simulink model "platooning_multiple_followers"  (R2018a)
settings: Solver=FixedStepAuto  StartTime=0.0  StopTime=70  FixedStep=timestep  RelTol=1e-3
model workspace (MAT data in the model file):
  t_0 = 0
undefined symbols (not defined in the file): a_max, a_min, canChannel, follower_1, follower_2, follower_3, leader, N
libraries: canlib x16, canmsglib x15, dspstat3 x3, dspindex x3, simulink x1
(part 1 of 2)
settings Model: Creator=s132652  LastModifiedBy=hugo
settings CodeAppCC: StateflowObjectComments=on
settings SimscapeCC: SimscapeNormalizeSystem=off

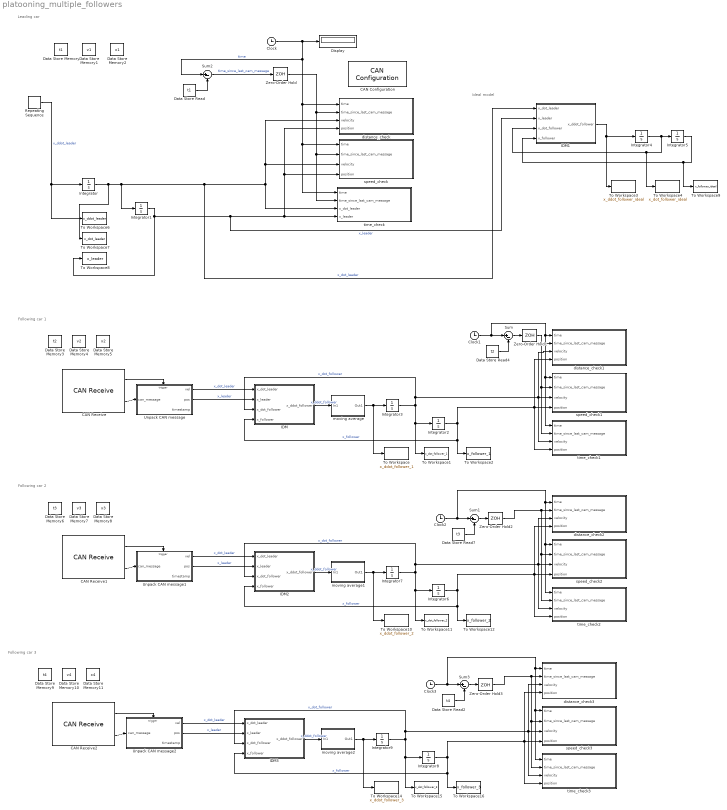
== system platooning_multiple_followers ==
  note: Ideal model
  note: Leading car
  note: Following car 1
  note: Following car 2
  note: Following car 3
  CAN Configuration : canlib/CAN Configuration  BlockHandle=4.0002  DeviceMenu=MathWorks Virtual 1 (Channel 1)  Device=MathWorks Virtual 1 (Channel 1)  ObjConstructor=canChannel('MathWorks','Virtual 1',1)  BusSpeed=500000  EnableBitParameters=off  SJW=0  TSEG1=0  TSEG2=0  NSamples=0  AckMode=Normal
      settings: SourceProductName=Vehicle Network Toolbox  SourceProductBaseCode=VN
  CAN Receive : canlib/CAN Receive  BlockHandle=5.0002  DeviceMenu=MathWorks Virtual 1 (Channel 1)  Device=MathWorks Virtual 1 (Channel 1)  ObjConstructor=canChannel('MathWorks','Virtual 1',1)  EnableStandardIDsFilter=off  StandardIDs=1  EnableExtendedIDsFilter=off  ExtendedIDs=0  SampleTime=0.001  MsgsPerTimestep=all  StdIDsCombo=Allow only  ExtIDsCombo=Allow all  InternalFilterUpdateStatus=on  BusOutput=off
      settings: SourceProductName=Vehicle Network Toolbox  SourceProductBaseCode=VN
  CAN Receive1 : canlib/CAN Receive  BlockHandle=6.0002  DeviceMenu=MathWorks Virtual 1 (Channel 1)  Device=MathWorks Virtual 1 (Channel 1)  ObjConstructor=canChannel('MathWorks','Virtual 1',1)  EnableStandardIDsFilter=off  StandardIDs=2  EnableExtendedIDsFilter=off  ExtendedIDs=0  SampleTime=0.001  MsgsPerTimestep=all  StdIDsCombo=Allow only  ExtIDsCombo=Allow all  InternalFilterUpdateStatus=on  BusOutput=off
      settings: SourceProductName=Vehicle Network Toolbox  SourceProductBaseCode=VN
  CAN Receive2 : canlib/CAN Receive  BlockHandle=7.0002  DeviceMenu=MathWorks Virtual 1 (Channel 1)  Device=MathWorks Virtual 1 (Channel 1)  ObjConstructor=canChannel('MathWorks','Virtual 1',1)  EnableStandardIDsFilter=off  StandardIDs=3  EnableExtendedIDsFilter=off  ExtendedIDs=0  SampleTime=0.001  MsgsPerTimestep=all  StdIDsCombo=Allow only  ExtIDsCombo=Allow all  InternalFilterUpdateStatus=on  BusOutput=off
      settings: SourceProductName=Vehicle Network Toolbox  SourceProductBaseCode=VN
  Clock{,1..3} (4 alike) : Clock
  Data Store Memory : DataStoreMemory  DataStoreName=t1  ReadBeforeWriteMsg=warning  WriteAfterWriteMsg=warning  WriteAfterReadMsg=warning  ShowAdditionalParam=off
  Data Store Memory1 : DataStoreMemory  DataStoreName=v1  ReadBeforeWriteMsg=warning  WriteAfterWriteMsg=warning  WriteAfterReadMsg=warning  InitialValue=leader.v0  ShowAdditionalParam=off
  Data Store Memory10 : DataStoreMemory  DataStoreName=v4  ReadBeforeWriteMsg=warning  WriteAfterWriteMsg=warning  WriteAfterReadMsg=warning  InitialValue=follower_3.v0  ShowAdditionalParam=off
  Data Store Memory11 : DataStoreMemory  DataStoreName=x4  ReadBeforeWriteMsg=warning  WriteAfterWriteMsg=warning  WriteAfterReadMsg=warning  InitialValue=follower_3.x0  ShowAdditionalParam=off
  Data Store Memory2 : DataStoreMemory  DataStoreName=x1  ReadBeforeWriteMsg=warning  WriteAfterWriteMsg=warning  WriteAfterReadMsg=warning  InitialValue=leader.x0  ShowAdditionalParam=off
  Data Store Memory3 : DataStoreMemory  DataStoreName=t2  ReadBeforeWriteMsg=warning  WriteAfterWriteMsg=warning  WriteAfterReadMsg=warning  ShowAdditionalParam=off
  Data Store Memory4 : DataStoreMemory  DataStoreName=v2  ReadBeforeWriteMsg=warning  WriteAfterWriteMsg=warning  WriteAfterReadMsg=warning  InitialValue=follower_1.v0  ShowAdditionalParam=off
  Data Store Memory5 : DataStoreMemory  DataStoreName=x2  ReadBeforeWriteMsg=warning  WriteAfterWriteMsg=warning  WriteAfterReadMsg=warning  InitialValue=follower_1.x0  ShowAdditionalParam=off
  Data Store Memory6 : DataStoreMemory  DataStoreName=t3  ReadBeforeWriteMsg=warning  WriteAfterWriteMsg=warning  WriteAfterReadMsg=warning  ShowAdditionalParam=off
  Data Store Memory7 : DataStoreMemory  DataStoreName=v3  ReadBeforeWriteMsg=warning  WriteAfterWriteMsg=warning  WriteAfterReadMsg=warning  InitialValue=follower_2.v0  ShowAdditionalParam=off
  Data Store Memory8 : DataStoreMemory  DataStoreName=x3  ReadBeforeWriteMsg=warning  WriteAfterWriteMsg=warning  WriteAfterReadMsg=warning  InitialValue=follower_2.x0  ShowAdditionalParam=off
  Data Store Memory9 : DataStoreMemory  DataStoreName=t4  ReadBeforeWriteMsg=warning  WriteAfterWriteMsg=warning  WriteAfterReadMsg=warning  ShowAdditionalParam=off
  Data Store Read : DataStoreRead  DataStoreName=t1
  Data Store Read2 : DataStoreRead  DataStoreName=t4
  Data Store Read4 : DataStoreRead  DataStoreName=t2
  Data Store Read7 : DataStoreRead  DataStoreName=t3
  Display : Display
  IDM : Subsystem
  IDM1 : Subsystem
  IDM2 : Subsystem
  IDM3 : Subsystem
  Integrator : Integrator  InitialCondition=leader.v0
  Integrator1 : Integrator  InitialCondition=leader.x0
  Integrator2 : Integrator  InitialCondition=follower_1.x0
  Integrator3 : Integrator  InitialCondition=follower_1.v0
  Integrator4 : Integrator  InitialCondition=follower_1.v0
  Integrator5 : Integrator  InitialCondition=follower_1.x0
  Integrator6 : Integrator  InitialCondition=follower_2.x0
  Integrator7 : Integrator  InitialCondition=follower_2.v0
  Integrator8 : Integrator  InitialCondition=follower_3.x0
  Integrator9 : Integrator  InitialCondition=follower_3.v0
  Repeating Sequence : simulink/Sources/Repeating Sequence  rep_seq_t=[0 5 10 15 20 25 30 35 40 45 50 55 60 65 70]  rep_seq_y=[0 0 0 0 0 a_max a_max 0 0 0 a_min a_min 0 0 0]
  Sum{,1..3} (4 alike) : Sum  Inputs=|+-
  To Workspace : ToWorkspace  VariableName=x_ddot_follower_1  SaveFormat=Timeseries  SampleTime=-1
  To Workspace1 : ToWorkspace  VariableName=x_dot_follower_1  SaveFormat=Timeseries  SampleTime=-1
  To Workspace10 : ToWorkspace  VariableName=x_ddot_follower_2  SaveFormat=Timeseries  SampleTime=-1
  To Workspace11 : ToWorkspace  VariableName=x_dot_follower_2  SaveFormat=Timeseries  SampleTime=-1
  To Workspace12 : ToWorkspace  VariableName=x_follower_2  SaveFormat=Timeseries  SampleTime=-1
  To Workspace14 : ToWorkspace  VariableName=x_ddot_follower_3  SaveFormat=Timeseries  SampleTime=-1
  To Workspace15 : ToWorkspace  VariableName=x_dot_follower_3  SaveFormat=Timeseries  SampleTime=-1
  To Workspace16 : ToWorkspace  VariableName=x_follower_3  SaveFormat=Timeseries  SampleTime=-1
  To Workspace2 : ToWorkspace  VariableName=x_follower_1  SaveFormat=Timeseries  SampleTime=-1
  To Workspace3 : ToWorkspace  VariableName=x_ddot_follower_ideal  SaveFormat=Timeseries  SampleTime=-1
  To Workspace4 : ToWorkspace  VariableName=x_dot_follower_ideal  SaveFormat=Timeseries  SampleTime=-1
  To Workspace6 : ToWorkspace  VariableName=x_ddot_leader  SaveFormat=Timeseries  SampleTime=-1
  To Workspace7 : ToWorkspace  VariableName=x_dot_leader  SaveFormat=Timeseries  SampleTime=-1
  To Workspace8 : ToWorkspace  VariableName=x_leader  SaveFormat=Timeseries  SampleTime=-1
  To Workspace9 : ToWorkspace  VariableName=x_follower_ideal  SaveFormat=Timeseries  SampleTime=-1
  Unpack CAN message : Subsystem  TreatAsAtomicUnit=on
  Unpack CAN message1 : Subsystem  TreatAsAtomicUnit=on
  Unpack CAN message2 : Subsystem  TreatAsAtomicUnit=on
  Zero-Order Hold{,1..3} (4 alike) : ZeroOrderHold  SampleTime=.001
  distance_check : Subsystem
  distance_check1 : Subsystem
  distance_check2 : Subsystem
  distance_check3 : Subsystem
  moving average : Subsystem
  moving average1 : Subsystem
  moving average2 : Subsystem
  speed_check : Subsystem
  speed_check1 : Subsystem
  speed_check2 : Subsystem
  speed_check3 : Subsystem
  time_check : Subsystem
  time_check1 : Subsystem
  time_check2 : Subsystem
  time_check3 : Subsystem
  wires:
  Repeating Sequence/1 -> To Workspace6/1, Integrator/1  "x_ddot_leader"
  Integrator/1 -> To Workspace7/1, Integrator1/1, IDM1/1(x_dot_leader), distance_check/3(velocity), speed_check/3(velocity), time_check/3(x_dot_leader)  "x_dot_leader"
  Integrator1/1 -> To Workspace8/1, IDM1/2(x_leader), distance_check/4(position), speed_check/4(position), time_check/4(x_leader)  "x_leader"
  Clock/1 -> time_check/1(time), speed_check/1(time), distance_check/1(time), Sum2/1, Display/1  "time"
  Data Store Read/1 -> Sum2/2
  Sum2/1 -> Zero-Order Hold/1  "time_since_last_cam_message"
  Zero-Order Hold/1 -> time_check/2(time_since_last_cam_message), speed_check/2(time_since_last_cam_message), distance_check/2(time_since_last_cam_message)
  CAN Receive/2 -> Unpack CAN message/1(can_message)
  CAN Receive/1 -> Unpack CAN message/Trigger
  Unpack CAN message/1(vel) -> IDM/1(x_dot_leader)  "x_dot_leader"
  Unpack CAN message/2(pos) -> IDM/2(x_leader)  "x_leader"
  IDM/1(x_ddot_follower) -> moving average/1(In1)  "x_ddot_follower"
  moving average/1(Out1) -> To Workspace/1, Integrator3/1
  Integrator3/1 -> speed_check1/3(velocity), distance_check1/3(velocity), time_check1/3(velocity), IDM/3(x_dot_follower), Integrator2/1, To Workspace1/1  "x_dot_follower"
  Integrator2/1 -> To Workspace2/1, IDM/4(x_follower), distance_check1/4(position), time_check1/4(position), speed_check1/4(position)  "x_follower"
  Integrator4/1 -> IDM1/3(x_dot_follower), To Workspace4/1, Integrator5/1
  Integrator5/1 -> IDM1/4(x_follower), To Workspace9/1
  IDM1/1(x_ddot_follower) -> Integrator4/1, To Workspace3/1
  Clock1/1 -> Sum/1, time_check1/1(time), speed_check1/1(time), distance_check1/1(time)
  Data Store Read4/1 -> Sum/2
  Sum/1 -> Zero-Order Hold1/1
  Zero-Order Hold1/1 -> time_check1/2(time_since_last_cam_message), speed_check1/2(time_since_last_cam_message), distance_check1/2(time_since_last_cam_message)
  Data Store Read7/1 -> Sum1/2
  Zero-Order Hold2/1 -> time_check2/2(time_since_last_cam_message), speed_check2/2(time_since_last_cam_message), distance_check2/2(time_since_last_cam_message)
  IDM2/1(x_ddot_follower) -> moving average1/1(In1)  "x_ddot_follower"
  Clock2/1 -> Sum1/1, time_check2/1(time), speed_check2/1(time), distance_check2/1(time)
  Integrator6/1 -> distance_check2/4(position), time_check2/4(position), speed_check2/4(position), To Workspace12/1, IDM2/4(x_follower)  "x_follower"
  Unpack CAN message1/2(pos) -> IDM2/2(x_leader)  "x_leader"
  Integrator7/1 -> speed_check2/3(velocity), distance_check2/3(velocity), time_check2/3(velocity), IDM2/3(x_dot_follower), Integrator6/1, To Workspace11/1  "x_dot_follower"
  moving average1/1(Out1) -> To Workspace10/1, Integrator7/1
  CAN Receive1/1 -> Unpack CAN message1/Trigger
  Unpack CAN message1/1(vel) -> IDM2/1(x_dot_leader)  "x_dot_leader"
  Sum1/1 -> Zero-Order Hold2/1
  CAN Receive1/2 -> Unpack CAN message1/1(can_message)
  Data Store Read2/1 -> Sum3/2
  CAN Receive2/1 -> Unpack CAN message2/Trigger
  IDM3/1(x_ddot_follower) -> moving average2/1(In1)  "x_ddot_follower"
  Sum3/1 -> Zero-Order Hold3/1
  CAN Receive2/2 -> Unpack CAN message2/1(can_message)
  Unpack CAN message2/1(vel) -> IDM3/1(x_dot_leader)  "x_dot_leader"
  Unpack CAN message2/2(pos) -> IDM3/2(x_leader)  "x_leader"
  Clock3/1 -> Sum3/1, time_check3/1(time), speed_check3/1(time), distance_check3/1(time)
  moving average2/1(Out1) -> To Workspace14/1, Integrator9/1
  Zero-Order Hold3/1 -> time_check3/2(time_since_last_cam_message), speed_check3/2(time_since_last_cam_message), distance_check3/2(time_since_last_cam_message)
  Integrator9/1 -> speed_check3/3(velocity), distance_check3/3(velocity), time_check3/3(velocity), IDM3/3(x_dot_follower), Integrator8/1, To Workspace15/1  "x_dot_follower"
  Integrator8/1 -> distance_check3/4(position), time_check3/4(position), speed_check3/4(position), To Workspace16/1, IDM3/4(x_follower)  "x_follower"

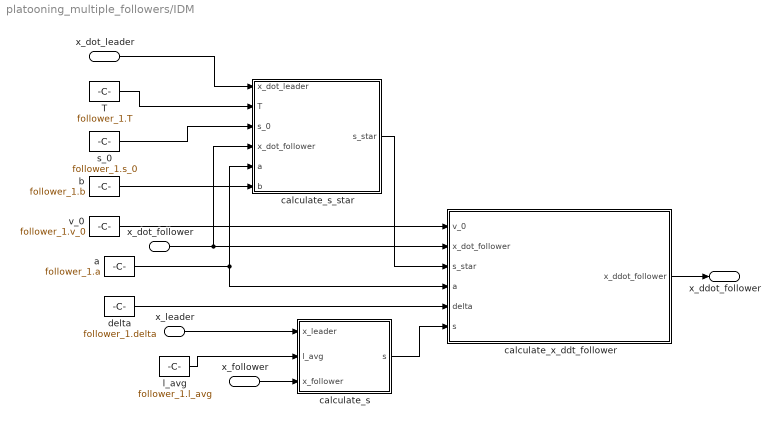
== system platooning_multiple_followers/IDM ==
  x_dot_leader : Inport
  x_leader : Inport  Port=2
  x_dot_follower : Inport  Port=3
  x_follower : Inport  Port=4
  T : Constant  Value=follower_1.T
  a : Constant  Value=follower_1.a
  b : Constant  Value=follower_1.b
  calculate_s : Subsystem
  calculate_s_star : Subsystem
  calculate_x_ddt_follower : Subsystem
  delta : Constant  Value=follower_1.delta
  l_avg : Constant  Value=follower_1.l_avg
  s_0 : Constant  Value=follower_1.s_0
  v_0 : Constant  Value=follower_1.v_0
  x_ddot_follower : Outport
  wires:
  v_0/1 -> calculate_x_ddt_follower/1(v_0)
  T/1 -> calculate_s_star/2(T)
  s_0/1 -> calculate_s_star/3(s_0)
  calculate_x_ddt_follower/1(x_ddot_follower) -> x_ddot_follower/1
  b/1 -> calculate_s_star/6(b)
  l_avg/1 -> calculate_s/2(l_avg)
  calculate_s/1(s) -> calculate_x_ddt_follower/6(s)
  delta/1 -> calculate_x_ddt_follower/5(delta)
  calculate_s_star/1(s_star) -> calculate_x_ddt_follower/3(s_star)
  x_follower/1 -> calculate_s/3(x_follower)
  x_dot_leader/1 -> calculate_s_star/1(x_dot_leader)
  x_leader/1 -> calculate_s/1(x_leader)
  x_dot_follower/1 -> calculate_s_star/4(x_dot_follower), calculate_x_ddt_follower/2(x_dot_follower)
  a/1 -> calculate_x_ddt_follower/4(a), calculate_s_star/5(a)

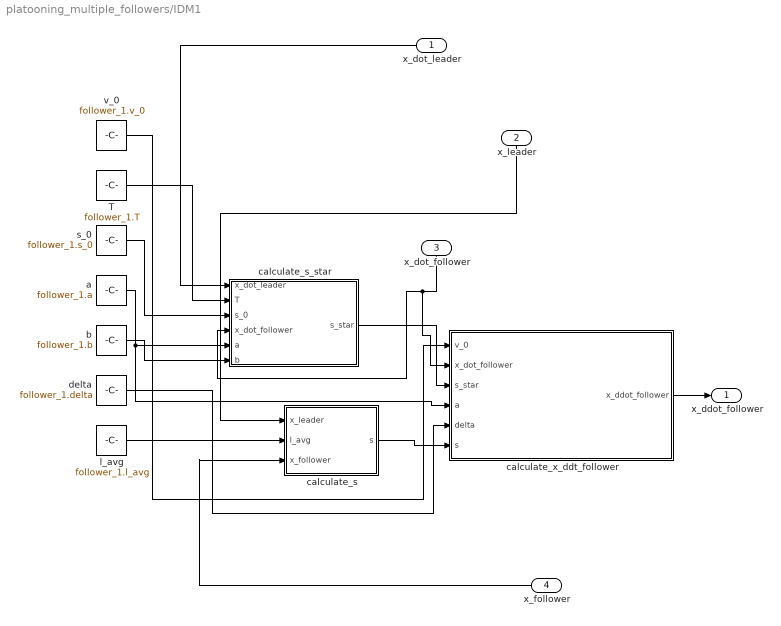
== system platooning_multiple_followers/IDM1 ==
  x_dot_leader : Inport
  x_leader : Inport  Port=2
  x_dot_follower : Inport  Port=3
  x_follower : Inport  Port=4
  T : Constant  Value=follower_1.T
  a : Constant  Value=follower_1.a
  b : Constant  Value=follower_1.b
  calculate_s : Subsystem
  calculate_s_star : Subsystem
  calculate_x_ddt_follower : Subsystem
  delta : Constant  Value=follower_1.delta
  l_avg : Constant  Value=follower_1.l_avg
  "s_0 " : Constant  Value=follower_1.s_0
  v_0 : Constant  Value=follower_1.v_0
  x_ddot_follower : Outport
  wires:
  a/1 -> calculate_x_ddt_follower/4(a), calculate_s_star/5(a)
  v_0/1 -> calculate_x_ddt_follower/1(v_0)
  T/1 -> calculate_s_star/2(T)
  "s_0 "/1 -> calculate_s_star/3(s_0)
  calculate_x_ddt_follower/1(x_ddot_follower) -> x_ddot_follower/1
  b/1 -> calculate_s_star/6(b)
  l_avg/1 -> calculate_s/2(l_avg)
  calculate_s/1(s) -> calculate_x_ddt_follower/6(s)
  delta/1 -> calculate_x_ddt_follower/5(delta)
  calculate_s_star/1(s_star) -> calculate_x_ddt_follower/3(s_star)
  x_follower/1 -> calculate_s/3(x_follower)
  x_dot_follower/1 -> calculate_x_ddt_follower/2(x_dot_follower), calculate_s_star/4(x_dot_follower)
  x_dot_leader/1 -> calculate_s_star/1(x_dot_leader)
  x_leader/1 -> calculate_s/1(x_leader)

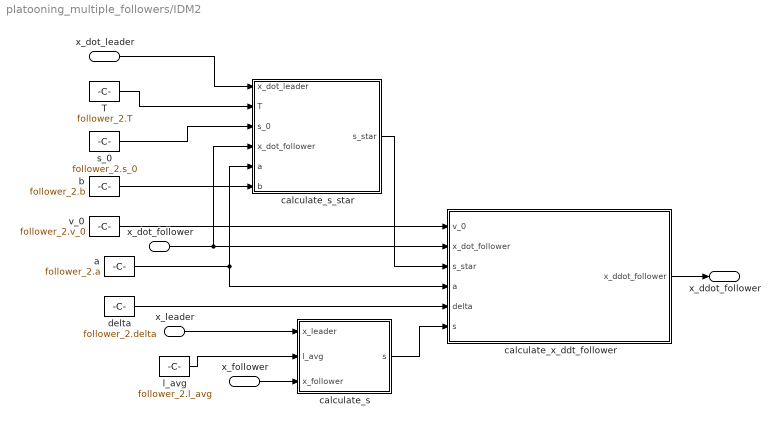
== system platooning_multiple_followers/IDM2 ==
  x_dot_leader : Inport
  x_leader : Inport  Port=2
  x_dot_follower : Inport  Port=3
  x_follower : Inport  Port=4
  T : Constant  Value=follower_2.T
  a : Constant  Value=follower_2.a
  b : Constant  Value=follower_2.b
  calculate_s : Subsystem
  calculate_s_star : Subsystem
  calculate_x_ddt_follower : Subsystem
  delta : Constant  Value=follower_2.delta
  l_avg : Constant  Value=follower_2.l_avg
  s_0 : Constant  Value=follower_2.s_0
  v_0 : Constant  Value=follower_2.v_0
  x_ddot_follower : Outport
  wires:
  v_0/1 -> calculate_x_ddt_follower/1(v_0)
  T/1 -> calculate_s_star/2(T)
  s_0/1 -> calculate_s_star/3(s_0)
  calculate_x_ddt_follower/1(x_ddot_follower) -> x_ddot_follower/1
  b/1 -> calculate_s_star/6(b)
  l_avg/1 -> calculate_s/2(l_avg)
  calculate_s/1(s) -> calculate_x_ddt_follower/6(s)
  delta/1 -> calculate_x_ddt_follower/5(delta)
  calculate_s_star/1(s_star) -> calculate_x_ddt_follower/3(s_star)
  x_follower/1 -> calculate_s/3(x_follower)
  x_dot_leader/1 -> calculate_s_star/1(x_dot_leader)
  x_leader/1 -> calculate_s/1(x_leader)
  x_dot_follower/1 -> calculate_s_star/4(x_dot_follower), calculate_x_ddt_follower/2(x_dot_follower)
  a/1 -> calculate_x_ddt_follower/4(a), calculate_s_star/5(a)

== system platooning_multiple_followers/IDM3 ==
  x_dot_leader : Inport
  x_leader : Inport  Port=2
  x_dot_follower : Inport  Port=3
  x_follower : Inport  Port=4
  T : Constant  Value=follower_3.T
  a : Constant  Value=follower_3.a
  b : Constant  Value=follower_3.b
  calculate_s : Subsystem
  calculate_s_star : Subsystem
  calculate_x_ddt_follower : Subsystem
  delta : Constant  Value=follower_3.delta
  l_avg : Constant  Value=follower_3.l_avg
  s_0 : Constant  Value=follower_3.s_0
  v_0 : Constant  Value=follower_3.v_0
  x_ddot_follower : Outport
  wires:
  v_0/1 -> calculate_x_ddt_follower/1(v_0)
  T/1 -> calculate_s_star/2(T)
  s_0/1 -> calculate_s_star/3(s_0)
  calculate_x_ddt_follower/1(x_ddot_follower) -> x_ddot_follower/1
  b/1 -> calculate_s_star/6(b)
  l_avg/1 -> calculate_s/2(l_avg)
  calculate_s/1(s) -> calculate_x_ddt_follower/6(s)
  delta/1 -> calculate_x_ddt_follower/5(delta)
  calculate_s_star/1(s_star) -> calculate_x_ddt_follower/3(s_star)
  x_follower/1 -> calculate_s/3(x_follower)
  x_dot_leader/1 -> calculate_s_star/1(x_dot_leader)
  x_leader/1 -> calculate_s/1(x_leader)
  x_dot_follower/1 -> calculate_s_star/4(x_dot_follower), calculate_x_ddt_follower/2(x_dot_follower)
  a/1 -> calculate_x_ddt_follower/4(a), calculate_s_star/5(a)

== system platooning_multiple_followers/Unpack CAN message ==
  can_message : Inport
  function : TriggerPort  TriggerType=function-call  VariantControl=Variant
  CAN Unpack : canmsglib/CAN Unpack  MsgList=(none)  MsgName=CAN Msg  MsgIDType=Standard (11-bit identifier)  MsgIdentifier=1  MsgLength=8  SignalInfo=position$0$16$1$1$1$0$0.1$0$-Inf$Inf$#velocity$16$16$1$1$1$0$0.0025$0$-Inf$Inf$#timestamp$32$16$1$1$1$0$0.01$0$-Inf$Inf$#  NSignals=3  IDPort=off  TimestampPort=off  ErrorPort=off  RemotePort=off  LengthPort=off  StatusPort=off  StartBits=str2num('[int32(0);int32(16);int32(32)]')  SignalSizes=str2num('[int32(16);int32(16);int32(16)]')  ByteOrders=str2num('[int32(1);int32(1);int32(1)]')  DataTypes=str2num('[int32(1);int32(1);int32(1)]')  MultiplexTypes=str2num('[int32(1);int32(1);int32(1)]')  MultiplexValues=str2num('[double(0);double(0);double(0)]')  Factors=str2num('[double(0.1);double(0.0025);double(0.01)]')  Offsets=str2num('[double(0);double(0);double(0)]')  Minimums=str2num('[double(-Inf);double(-Inf);double(-Inf)]')  Maximums=str2num('[double(Inf);double(Inf);double(Inf)]')  ApplyMinMax=off
      settings: SourceProductName=Simulink Real-Time
  vel : Outport
  pos : Outport  Port=2
  timestamp : Outport  Port=3
  wires:
  can_message/1 -> CAN Unpack/1
  CAN Unpack/2 -> vel/1
  CAN Unpack/1 -> pos/1
  CAN Unpack/3 -> timestamp/1

== system platooning_multiple_followers/Unpack CAN message1 ==
  can_message : Inport
  function : TriggerPort  TriggerType=function-call  VariantControl=Variant
  CAN Unpack : canmsglib/CAN Unpack  MsgList=(none)  MsgName=CAN Msg  MsgIDType=Standard (11-bit identifier)  MsgIdentifier=2  MsgLength=8  SignalInfo=position$0$16$1$1$1$0$0.1$0$-Inf$Inf$#velocity$16$16$1$1$1$0$0.0025$0$-Inf$Inf$#timestamp$32$16$1$1$1$0$0.01$0$-Inf$Inf$#  NSignals=3  IDPort=off  TimestampPort=off  ErrorPort=off  RemotePort=off  LengthPort=off  StatusPort=off  StartBits=str2num('[int32(0);int32(16);int32(32)]')  SignalSizes=str2num('[int32(16);int32(16);int32(16)]')  ByteOrders=str2num('[int32(1);int32(1);int32(1)]')  DataTypes=str2num('[int32(1);int32(1);int32(1)]')  MultiplexTypes=str2num('[int32(1);int32(1);int32(1)]')  MultiplexValues=str2num('[double(0);double(0);double(0)]')  Factors=str2num('[double(0.1);double(0.0025);double(0.01)]')  Offsets=str2num('[double(0);double(0);double(0)]')  Minimums=str2num('[double(-Inf);double(-Inf);double(-Inf)]')  Maximums=str2num('[double(Inf);double(Inf);double(Inf)]')  ApplyMinMax=off
      settings: SourceProductName=Simulink Real-Time
  vel : Outport
  pos : Outport  Port=2
  timestamp : Outport  Port=3
  wires:
  can_message/1 -> CAN Unpack/1
  CAN Unpack/2 -> vel/1
  CAN Unpack/1 -> pos/1
  CAN Unpack/3 -> timestamp/1

== system platooning_multiple_followers/Unpack CAN message2 ==
  can_message : Inport
  function : TriggerPort  TriggerType=function-call  VariantControl=Variant
  CAN Unpack : canmsglib/CAN Unpack  MsgList=(none)  MsgName=CAN Msg  MsgIDType=Standard (11-bit identifier)  MsgIdentifier=3  MsgLength=8  SignalInfo=position$0$16$1$1$1$0$0.1$0$-Inf$Inf$#velocity$16$16$1$1$1$0$0.0025$0$-Inf$Inf$#timestamp$32$16$1$1$1$0$0.01$0$-Inf$Inf$#  NSignals=3  IDPort=off  TimestampPort=off  ErrorPort=off  RemotePort=off  LengthPort=off  StatusPort=off  StartBits=str2num('[int32(0);int32(16);int32(32)]')  SignalSizes=str2num('[int32(16);int32(16);int32(16)]')  ByteOrders=str2num('[int32(1);int32(1);int32(1)]')  DataTypes=str2num('[int32(1);int32(1);int32(1)]')  MultiplexTypes=str2num('[int32(1);int32(1);int32(1)]')  MultiplexValues=str2num('[double(0);double(0);double(0)]')  Factors=str2num('[double(0.1);double(0.0025);double(0.01)]')  Offsets=str2num('[double(0);double(0);double(0)]')  Minimums=str2num('[double(-Inf);double(-Inf);double(-Inf)]')  Maximums=str2num('[double(Inf);double(Inf);double(Inf)]')  ApplyMinMax=off
      settings: SourceProductName=Simulink Real-Time
  vel : Outport
  pos : Outport  Port=2
  timestamp : Outport  Port=3
  wires:
  can_message/1 -> CAN Unpack/1
  CAN Unpack/2 -> vel/1
  CAN Unpack/1 -> pos/1
  CAN Unpack/3 -> timestamp/1

== system platooning_multiple_followers/distance_check ==
  time : Inport
  time_since_last_cam_message : Inport  Port=2
  velocity : Inport  Port=3
  position : Inport  Port=4
  Abs1 : Abs
  Data Store Read3 : DataStoreRead  DataStoreName=x1
  If Action Subsystem2 : Subsystem  TreatAsAtomicUnit=on
  If2 : If  NumInputs=2  IfExpression=u1 >= D_THRESHOLD & u2 >= 0.1
  Sum1 : Sum  Inputs=|+-
  Zero-Order Hold2 : ZeroOrderHold  SampleTime=.001
  wires:
  Data Store Read3/1 -> Sum1/2
  Sum1/1 -> Abs1/1
  Abs1/1 -> Zero-Order Hold2/1
  Zero-Order Hold2/1 -> If2/1
  If2/1 -> If Action Subsystem2/Action
  time_since_last_cam_message/1 -> If2/2
  time/1 -> If Action Subsystem2/1(time)
  position/1 -> If Action Subsystem2/3(position), Sum1/1
  velocity/1 -> If Action Subsystem2/2(velocity)

== system platooning_multiple_followers/distance_check1 ==
  time : Inport
  time_since_last_cam_message : Inport  Port=2
  velocity : Inport  Port=3
  position : Inport  Port=4
  Abs1 : Abs
  Data Store Read3 : DataStoreRead  DataStoreName=x2
  If Action Subsystem2 : Subsystem  TreatAsAtomicUnit=on
  If2 : If  NumInputs=2  IfExpression=u1 >= D_THRESHOLD & u2 >= 0.1
  Sum1 : Sum  Inputs=|+-
  Zero-Order Hold2 : ZeroOrderHold  SampleTime=.001
  wires:
  Data Store Read3/1 -> Sum1/2
  Sum1/1 -> Abs1/1
  Abs1/1 -> Zero-Order Hold2/1
  Zero-Order Hold2/1 -> If2/1
  If2/1 -> If Action Subsystem2/Action
  time_since_last_cam_message/1 -> If2/2
  time/1 -> If Action Subsystem2/1(time)
  position/1 -> If Action Subsystem2/3(position), Sum1/1
  velocity/1 -> If Action Subsystem2/2(velocity)

== system platooning_multiple_followers/distance_check2 ==
  time : Inport
  time_since_last_cam_message : Inport  Port=2
  velocity : Inport  Port=3
  position : Inport  Port=4
  Abs1 : Abs
  Data Store Read3 : DataStoreRead  DataStoreName=x3
  If Action Subsystem2 : Subsystem  TreatAsAtomicUnit=on
  If2 : If  NumInputs=2  IfExpression=u1 >= D_THRESHOLD & u2 >= 0.1
  Sum1 : Sum  Inputs=|+-
  Zero-Order Hold2 : ZeroOrderHold  SampleTime=.001
  wires:
  Data Store Read3/1 -> Sum1/2
  Sum1/1 -> Abs1/1
  Abs1/1 -> Zero-Order Hold2/1
  Zero-Order Hold2/1 -> If2/1
  If2/1 -> If Action Subsystem2/Action
  time_since_last_cam_message/1 -> If2/2
  time/1 -> If Action Subsystem2/1(time)
  position/1 -> If Action Subsystem2/3(position), Sum1/1
  velocity/1 -> If Action Subsystem2/2(velocity)

== system platooning_multiple_followers/distance_check3 ==
  time : Inport
  time_since_last_cam_message : Inport  Port=2
  velocity : Inport  Port=3
  position : Inport  Port=4
  Abs1 : Abs
  Data Store Read3 : DataStoreRead  DataStoreName=x4
  If Action Subsystem2 : Subsystem  TreatAsAtomicUnit=on
  If2 : If  NumInputs=2  IfExpression=u1 >= D_THRESHOLD & u2 >= 0.1
  Sum1 : Sum  Inputs=|+-
  Zero-Order Hold2 : ZeroOrderHold  SampleTime=.001
  wires:
  Data Store Read3/1 -> Sum1/2
  Sum1/1 -> Abs1/1
  Abs1/1 -> Zero-Order Hold2/1
  Zero-Order Hold2/1 -> If2/1
  If2/1 -> If Action Subsystem2/Action
  time_since_last_cam_message/1 -> If2/2
  time/1 -> If Action Subsystem2/1(time)
  position/1 -> If Action Subsystem2/3(position), Sum1/1
  velocity/1 -> If Action Subsystem2/2(velocity)

== system platooning_multiple_followers/moving average ==
  note: moving average
  In1 : Inport
  IC : InitialCondition  Value=zeros(N,1)
  Mean : dspstat3/Mean  run=off  InputProcessing=Columns as channels (frame based)  reset_popup=None  directionMode=Each column  dimension=1  roiEnable=off  roiType=Rectangles  roiPortion=Entire ROI  roiOutput=Individual statistics for each ROI  roiFlag=off  roundingMode=Floor  overflowMode=off  outputDataTypeStr=Inherit: Same as accumulator  outputMin=[]  outputMax=[]  outputLastDataTypeStr=Inherit: Same as accumulator
  Memory : Memory
  Mux : Mux  Inputs=2
  Variable Selector : dspindex/Variable Selector  NumInputs=1  rowsOrCols=Rows  IdxMode=Fixed  Elements=1:N-1  ZerOneIdxMode=One-based  errmode=Clip Index  FillMode=on  FillValues=0
  Out1 : Outport
  wires:
  In1/1 -> Mux/1
  Mux/1 -> Mean/1, Memory/1
  Memory/1 -> IC/1
  IC/1 -> Variable Selector/1
  Mean/1 -> Out1/1
  Variable Selector/1 -> Mux/2

== system platooning_multiple_followers/moving average1 ==
  note: moving average
  In1 : Inport
  IC : InitialCondition  Value=zeros(N,1)
  Mean : dspstat3/Mean  run=off  InputProcessing=Columns as channels (frame based)  reset_popup=None  directionMode=Each column  dimension=1  roiEnable=off  roiType=Rectangles  roiPortion=Entire ROI  roiOutput=Individual statistics for each ROI  roiFlag=off  roundingMode=Floor  overflowMode=off  outputDataTypeStr=Inherit: Same as accumulator  outputMin=[]  outputMax=[]  outputLastDataTypeStr=Inherit: Same as accumulator
  Memory : Memory
  Mux : Mux  Inputs=2
  Variable Selector : dspindex/Variable Selector  NumInputs=1  rowsOrCols=Rows  IdxMode=Fixed  Elements=1:N-1  ZerOneIdxMode=One-based  errmode=Clip Index  FillMode=on  FillValues=0
  Out1 : Outport
  wires:
  In1/1 -> Mux/1
  Mux/1 -> Mean/1, Memory/1
  Memory/1 -> IC/1
  IC/1 -> Variable Selector/1
  Mean/1 -> Out1/1
  Variable Selector/1 -> Mux/2

== system platooning_multiple_followers/moving average2 ==
  note: moving average
  In1 : Inport
  IC : InitialCondition  Value=zeros(N,1)
  Mean : dspstat3/Mean  run=off  InputProcessing=Columns as channels (frame based)  reset_popup=None  directionMode=Each column  dimension=1  roiEnable=off  roiType=Rectangles  roiPortion=Entire ROI  roiOutput=Individual statistics for each ROI  roiFlag=off  roundingMode=Floor  overflowMode=off  outputDataTypeStr=Inherit: Same as accumulator  outputMin=[]  outputMax=[]  outputLastDataTypeStr=Inherit: Same as accumulator
  Memory : Memory
  Mux : Mux  Inputs=2
  Variable Selector : dspindex/Variable Selector  NumInputs=1  rowsOrCols=Rows  IdxMode=Fixed  Elements=1:N-1  ZerOneIdxMode=One-based  errmode=Clip Index  FillMode=on  FillValues=0
  Out1 : Outport
  wires:
  In1/1 -> Mux/1
  Mux/1 -> Mean/1, Memory/1
  Memory/1 -> IC/1
  IC/1 -> Variable Selector/1
  Mean/1 -> Out1/1
  Variable Selector/1 -> Mux/2

== system platooning_multiple_followers/speed_check ==
  time : Inport
  time_since_last_cam_message : Inport  Port=2
  velocity : Inport  Port=3
  position : Inport  Port=4
  Abs : Abs
  Data Store Read2 : DataStoreRead  DataStoreName=v1
  If Action Subsystem1 : Subsystem  TreatAsAtomicUnit=on
  If1 : If  NumInputs=2  IfExpression=u1 >= S_THRESHOLD & u2 >= 0.1
  Sum : Sum  Inputs=|+-
  Zero-Order Hold1 : ZeroOrderHold  SampleTime=.001
  wires:
  Data Store Read2/1 -> Sum/2
  Sum/1 -> Abs/1
  Abs/1 -> Zero-Order Hold1/1
  If1/1 -> If Action Subsystem1/Action
  Zero-Order Hold1/1 -> If1/1
  time/1 -> If Action Subsystem1/1(time)
  velocity/1 -> Sum/1, If Action Subsystem1/2(velocity)
  position/1 -> If Action Subsystem1/3(position)
  time_since_last_cam_message/1 -> If1/2

== system platooning_multiple_followers/speed_check1 ==
  time : Inport
  time_since_last_cam_message : Inport  Port=2
  velocity : Inport  Port=3
  position : Inport  Port=4
  Abs : Abs
  Data Store Read2 : DataStoreRead  DataStoreName=v2
  If Action Subsystem1 : Subsystem  TreatAsAtomicUnit=on
  If1 : If  NumInputs=2  IfExpression=u1 >= S_THRESHOLD & u2 >= 0.1
  Sum : Sum  Inputs=|+-
  Zero-Order Hold1 : ZeroOrderHold  SampleTime=.001
  wires:
  Data Store Read2/1 -> Sum/2
  Sum/1 -> Abs/1
  Abs/1 -> Zero-Order Hold1/1
  If1/1 -> If Action Subsystem1/Action
  Zero-Order Hold1/1 -> If1/1
  time/1 -> If Action Subsystem1/1(time)
  velocity/1 -> Sum/1, If Action Subsystem1/2(velocity)
  position/1 -> If Action Subsystem1/3(position)
  time_since_last_cam_message/1 -> If1/2

== system platooning_multiple_followers/speed_check2 ==
  time : Inport
  time_since_last_cam_message : Inport  Port=2
  velocity : Inport  Port=3
  position : Inport  Port=4
  Abs : Abs
  Data Store Read2 : DataStoreRead  DataStoreName=v3
  If Action Subsystem1 : Subsystem  TreatAsAtomicUnit=on
  If1 : If  NumInputs=2  IfExpression=u1 >= S_THRESHOLD & u2 >= 0.1
  Sum : Sum  Inputs=|+-
  Zero-Order Hold1 : ZeroOrderHold  SampleTime=.001
  wires:
  Data Store Read2/1 -> Sum/2
  Sum/1 -> Abs/1
  Abs/1 -> Zero-Order Hold1/1
  If1/1 -> If Action Subsystem1/Action
  Zero-Order Hold1/1 -> If1/1
  time/1 -> If Action Subsystem1/1(time)
  velocity/1 -> Sum/1, If Action Subsystem1/2(velocity)
  position/1 -> If Action Subsystem1/3(position)
  time_since_last_cam_message/1 -> If1/2

== system platooning_multiple_followers/speed_check3 ==
  time : Inport
  time_since_last_cam_message : Inport  Port=2
  velocity : Inport  Port=3
  position : Inport  Port=4
  Abs : Abs
  Data Store Read2 : DataStoreRead  DataStoreName=v4
  If Action Subsystem1 : Subsystem  TreatAsAtomicUnit=on
  If1 : If  NumInputs=2  IfExpression=u1 >= S_THRESHOLD & u2 >= 0.1
  Sum : Sum  Inputs=|+-
  Zero-Order Hold1 : ZeroOrderHold  SampleTime=.001
  wires:
  Data Store Read2/1 -> Sum/2
  Sum/1 -> Abs/1
  Abs/1 -> Zero-Order Hold1/1
  If1/1 -> If Action Subsystem1/Action
  Zero-Order Hold1/1 -> If1/1
  time/1 -> If Action Subsystem1/1(time)
  velocity/1 -> Sum/1, If Action Subsystem1/2(velocity)
  position/1 -> If Action Subsystem1/3(position)
  time_since_last_cam_message/1 -> If1/2

== system platooning_multiple_followers/time_check ==
  time : Inport
  time_since_last_cam_message : Inport  Port=2
  x_dot_leader : Inport  Port=3
  x_leader : Inport  Port=4
  If : If  IfExpression=u1 >= T_THRESHOLD
  If Action Subsystem : Subsystem  TreatAsAtomicUnit=on
  wires:
  If/1 -> If Action Subsystem/Action
  time_since_last_cam_message/1 -> If/1
  time/1 -> If Action Subsystem/1(time)
  x_dot_leader/1 -> If Action Subsystem/2(velocity)
  x_leader/1 -> If Action Subsystem/3(position)

== system platooning_multiple_followers/time_check1 ==
  time : Inport
  time_since_last_cam_message : Inport  Port=2
  velocity : Inport  Port=3
  position : Inport  Port=4
  If : If  IfExpression=u1 >= T_THRESHOLD
  If Action Subsystem : Subsystem  TreatAsAtomicUnit=on
  wires:
  If/1 -> If Action Subsystem/Action
  time_since_last_cam_message/1 -> If/1
  time/1 -> If Action Subsystem/1(time)
  velocity/1 -> If Action Subsystem/2(velocity)
  position/1 -> If Action Subsystem/3(position)

== system platooning_multiple_followers/time_check2 ==
  time : Inport
  time_since_last_cam_message : Inport  Port=2
  velocity : Inport  Port=3
  position : Inport  Port=4
  If : If  IfExpression=u1 >= T_THRESHOLD
  If Action Subsystem : Subsystem  TreatAsAtomicUnit=on
  wires:
  If/1 -> If Action Subsystem/Action
  time_since_last_cam_message/1 -> If/1
  time/1 -> If Action Subsystem/1(time)
  velocity/1 -> If Action Subsystem/2(velocity)
  position/1 -> If Action Subsystem/3(position)

== system platooning_multiple_followers/time_check3 ==
  time : Inport
  time_since_last_cam_message : Inport  Port=2
  velocity : Inport  Port=3
  position : Inport  Port=4
  If : If  IfExpression=u1 >= T_THRESHOLD
  If Action Subsystem : Subsystem  TreatAsAtomicUnit=on
  wires:
  If/1 -> If Action Subsystem/Action
  time_since_last_cam_message/1 -> If/1
  time/1 -> If Action Subsystem/1(time)
  velocity/1 -> If Action Subsystem/2(velocity)
  position/1 -> If Action Subsystem/3(position)

== system platooning_multiple_followers/IDM/calculate_s ==
  x_leader : Inport
  l_avg : Inport  Port=2
  x_follower : Inport  Port=3
  Sum3 : Sum  Inputs=|+-
  Sum4 : Sum  Inputs=|+-
  s : Outport
  wires:
  Sum4/1 -> s/1  "s"
  Sum3/1 -> Sum4/1
  l_avg/1 -> Sum4/2
  x_follower/1 -> Sum3/2
  x_leader/1 -> Sum3/1

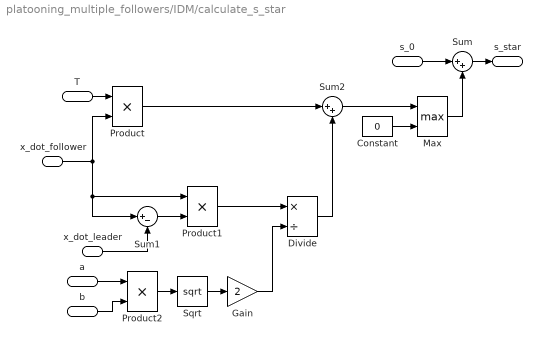
== system platooning_multiple_followers/IDM/calculate_s_star ==
  x_dot_leader : Inport
  T : Inport  Port=2
  s_0 : Inport  Port=3
  x_dot_follower : Inport  Port=4
  a : Inport  Port=5
  b : Inport  Port=6
  Constant : Constant  Value=0
  Divide : Product  Inputs=*/
  Gain : Gain  Gain=2
  Max : MinMax  Function=max  Inputs=2
  Product : Product
  Product1 : Product
  Product2 : Product
  Sqrt : Sqrt  SaturateOnIntegerOverflow=on
  Sum : Sum  Inputs=|++
  Sum1 : Sum  Inputs=|+-
  Sum2 : Sum  Inputs=|++
  s_star : Outport
  wires:
  Sum1/1 -> Product1/2
  T/1 -> Product/1
  s_0/1 -> Sum/1
  Product1/1 -> Divide/1
  Product/1 -> Sum2/1
  Divide/1 -> Sum2/2
  x_dot_leader/1 -> Sum1/2
  Product2/1 -> Sqrt/1
  Sqrt/1 -> Gain/1
  Gain/1 -> Divide/2
  a/1 -> Product2/1
  b/1 -> Product2/2
  Constant/1 -> Max/2
  Sum2/1 -> Max/1
  Max/1 -> Sum/2
  Sum/1 -> s_star/1
  x_dot_follower/1 -> Product/2, Product1/1, Sum1/1

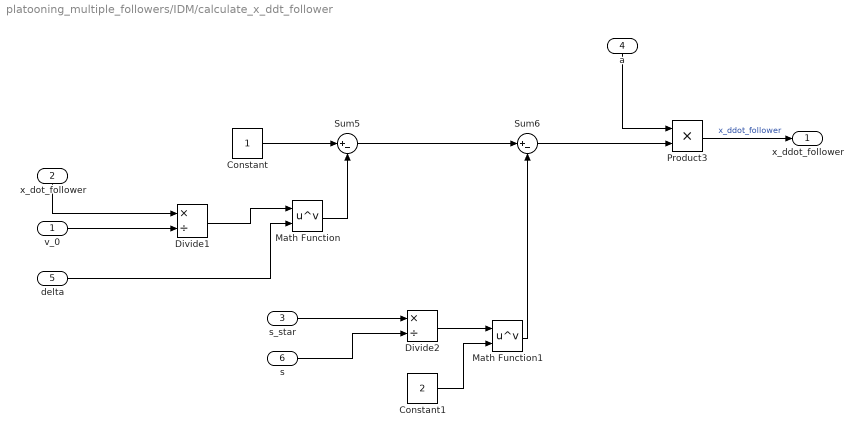
== system platooning_multiple_followers/IDM/calculate_x_ddt_follower ==
  v_0 : Inport
  x_dot_follower : Inport  Port=2
  s_star : Inport  Port=3
  a : Inport  Port=4
  delta : Inport  Port=5
  s : Inport  Port=6
  Constant : Constant
  Constant1 : Constant  Value=2
  Divide1 : Product  Inputs=*/
  Divide2 : Product  Inputs=*/
  Math Function : Math  Operator=pow  SaturateOnIntegerOverflow=on
  Math Function1 : Math  Operator=pow  SaturateOnIntegerOverflow=on
  Product3 : Product
  Sum5 : Sum  Inputs=|+-
  Sum6 : Sum  Inputs=|+-
  x_ddot_follower : Outport
  wires:
  Product3/1 -> x_ddot_follower/1  "x_ddot_follower"
  v_0/1 -> Divide1/2
  Constant/1 -> Sum5/1
  Math Function/1 -> Sum5/2
  a/1 -> Product3/1
  x_dot_follower/1 -> Divide1/1
  s/1 -> Divide2/2
  s_star/1 -> Divide2/1
  Sum5/1 -> Sum6/1
  Constant1/1 -> Math Function1/2
  Divide1/1 -> Math Function/1
  Math Function1/1 -> Sum6/2
  delta/1 -> Math Function/2
  Divide2/1 -> Math Function1/1
  Sum6/1 -> Product3/2

== system platooning_multiple_followers/IDM1/calculate_s ==
  x_leader : Inport
  l_avg : Inport  Port=2
  x_follower : Inport  Port=3
  Sum3 : Sum  Inputs=|+-
  Sum4 : Sum  Inputs=|+-
  s : Outport
  wires:
  Sum4/1 -> s/1  "s"
  Sum3/1 -> Sum4/1
  l_avg/1 -> Sum4/2
  x_follower/1 -> Sum3/2
  x_leader/1 -> Sum3/1

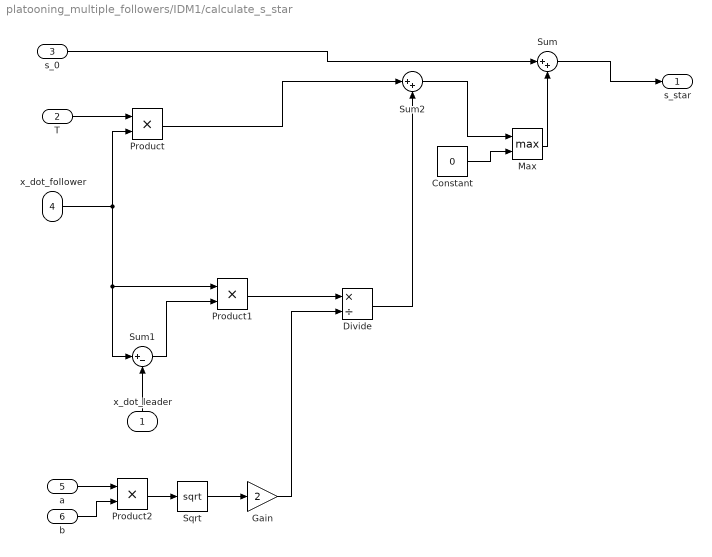
== system platooning_multiple_followers/IDM1/calculate_s_star ==
  x_dot_leader : Inport
  T : Inport  Port=2
  s_0 : Inport  Port=3
  x_dot_follower : Inport  Port=4
  a : Inport  Port=5
  b : Inport  Port=6
  Constant : Constant  Value=0
  Divide : Product  Inputs=*/
  Gain : Gain  Gain=2
  Max : MinMax  Function=max  Inputs=2
  Product : Product
  Product1 : Product
  Product2 : Product
  Sqrt : Sqrt  SaturateOnIntegerOverflow=on
  Sum : Sum  Inputs=|++
  Sum1 : Sum  Inputs=|+-
  Sum2 : Sum  Inputs=|++
  s_star : Outport
  wires:
  Sum1/1 -> Product1/2
  T/1 -> Product/1
  s_0/1 -> Sum/1
  Product1/1 -> Divide/1
  Product/1 -> Sum2/1
  Divide/1 -> Sum2/2
  x_dot_leader/1 -> Sum1/2
  x_dot_follower/1 -> Product/2, Sum1/1, Product1/1
  Product2/1 -> Sqrt/1
  Sqrt/1 -> Gain/1
  Gain/1 -> Divide/2
  a/1 -> Product2/1
  b/1 -> Product2/2
  Constant/1 -> Max/2
  Sum2/1 -> Max/1
  Max/1 -> Sum/2
  Sum/1 -> s_star/1

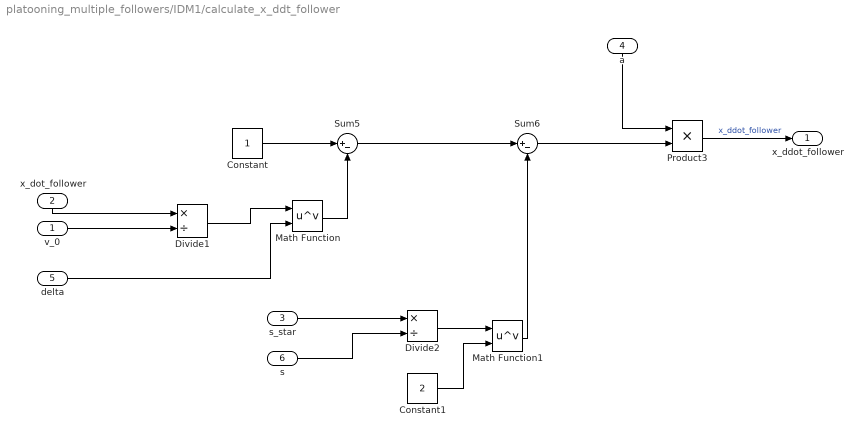
== system platooning_multiple_followers/IDM1/calculate_x_ddt_follower ==
  v_0 : Inport
  x_dot_follower : Inport  Port=2
  s_star : Inport  Port=3
  a : Inport  Port=4
  delta : Inport  Port=5
  s : Inport  Port=6
  Constant : Constant
  Constant1 : Constant  Value=2
  Divide1 : Product  Inputs=*/
  Divide2 : Product  Inputs=*/
  Math Function : Math  Operator=pow  SaturateOnIntegerOverflow=on
  Math Function1 : Math  Operator=pow  SaturateOnIntegerOverflow=on
  Product3 : Product
  Sum5 : Sum  Inputs=|+-
  Sum6 : Sum  Inputs=|+-
  x_ddot_follower : Outport
  wires:
  Product3/1 -> x_ddot_follower/1  "x_ddot_follower"
  v_0/1 -> Divide1/2
  Constant/1 -> Sum5/1
  Math Function/1 -> Sum5/2
  a/1 -> Product3/1
  x_dot_follower/1 -> Divide1/1
  s/1 -> Divide2/2
  s_star/1 -> Divide2/1
  Sum5/1 -> Sum6/1
  Constant1/1 -> Math Function1/2
  Divide1/1 -> Math Function/1
  Math Function1/1 -> Sum6/2
  delta/1 -> Math Function/2
  Divide2/1 -> Math Function1/1
  Sum6/1 -> Product3/2

== system platooning_multiple_followers/IDM2/calculate_s ==
  x_leader : Inport
  l_avg : Inport  Port=2
  x_follower : Inport  Port=3
  Sum3 : Sum  Inputs=|+-
  Sum4 : Sum  Inputs=|+-
  s : Outport
  wires:
  Sum4/1 -> s/1  "s"
  Sum3/1 -> Sum4/1
  l_avg/1 -> Sum4/2
  x_follower/1 -> Sum3/2
  x_leader/1 -> Sum3/1

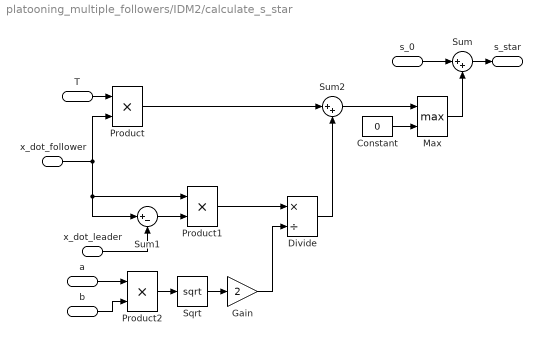
== system platooning_multiple_followers/IDM2/calculate_s_star ==
  x_dot_leader : Inport
  T : Inport  Port=2
  s_0 : Inport  Port=3
  x_dot_follower : Inport  Port=4
  a : Inport  Port=5
  b : Inport  Port=6
  Constant : Constant  Value=0
  Divide : Product  Inputs=*/
  Gain : Gain  Gain=2
  Max : MinMax  Function=max  Inputs=2
  Product : Product
  Product1 : Product
  Product2 : Product
  Sqrt : Sqrt  SaturateOnIntegerOverflow=on
  Sum : Sum  Inputs=|++
  Sum1 : Sum  Inputs=|+-
  Sum2 : Sum  Inputs=|++
  s_star : Outport
  wires:
  Sum1/1 -> Product1/2
  T/1 -> Product/1
  s_0/1 -> Sum/1
  Product1/1 -> Divide/1
  Product/1 -> Sum2/1
  Divide/1 -> Sum2/2
  x_dot_leader/1 -> Sum1/2
  Product2/1 -> Sqrt/1
  Sqrt/1 -> Gain/1
  Gain/1 -> Divide/2
  a/1 -> Product2/1
  b/1 -> Product2/2
  Constant/1 -> Max/2
  Sum2/1 -> Max/1
  Max/1 -> Sum/2
  Sum/1 -> s_star/1
  x_dot_follower/1 -> Product/2, Product1/1, Sum1/1

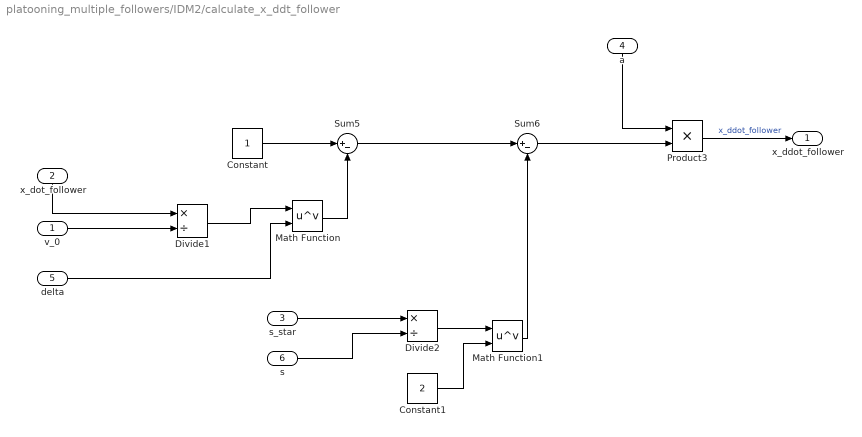
== system platooning_multiple_followers/IDM2/calculate_x_ddt_follower ==
  v_0 : Inport
  x_dot_follower : Inport  Port=2
  s_star : Inport  Port=3
  a : Inport  Port=4
  delta : Inport  Port=5
  s : Inport  Port=6
  Constant : Constant
  Constant1 : Constant  Value=2
  Divide1 : Product  Inputs=*/
  Divide2 : Product  Inputs=*/
  Math Function : Math  Operator=pow  SaturateOnIntegerOverflow=on
  Math Function1 : Math  Operator=pow  SaturateOnIntegerOverflow=on
  Product3 : Product
  Sum5 : Sum  Inputs=|+-
  Sum6 : Sum  Inputs=|+-
  x_ddot_follower : Outport
  wires:
  Product3/1 -> x_ddot_follower/1  "x_ddot_follower"
  v_0/1 -> Divide1/2
  Constant/1 -> Sum5/1
  Math Function/1 -> Sum5/2
  a/1 -> Product3/1
  x_dot_follower/1 -> Divide1/1
  s/1 -> Divide2/2
  s_star/1 -> Divide2/1
  Sum5/1 -> Sum6/1
  Constant1/1 -> Math Function1/2
  Divide1/1 -> Math Function/1
  Math Function1/1 -> Sum6/2
  delta/1 -> Math Function/2
  Divide2/1 -> Math Function1/1
  Sum6/1 -> Product3/2

== system platooning_multiple_followers/IDM3/calculate_s ==
  x_leader : Inport
  l_avg : Inport  Port=2
  x_follower : Inport  Port=3
  Sum3 : Sum  Inputs=|+-
  Sum4 : Sum  Inputs=|+-
  s : Outport
  wires:
  Sum4/1 -> s/1  "s"
  Sum3/1 -> Sum4/1
  l_avg/1 -> Sum4/2
  x_follower/1 -> Sum3/2
  x_leader/1 -> Sum3/1

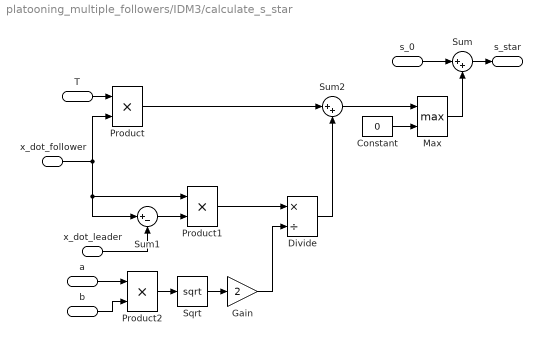
== system platooning_multiple_followers/IDM3/calculate_s_star ==
  x_dot_leader : Inport
  T : Inport  Port=2
  s_0 : Inport  Port=3
  x_dot_follower : Inport  Port=4
  a : Inport  Port=5
  b : Inport  Port=6
  Constant : Constant  Value=0
  Divide : Product  Inputs=*/
  Gain : Gain  Gain=2
  Max : MinMax  Function=max  Inputs=2
  Product : Product
  Product1 : Product
  Product2 : Product
  Sqrt : Sqrt  SaturateOnIntegerOverflow=on
  Sum : Sum  Inputs=|++
  Sum1 : Sum  Inputs=|+-
  Sum2 : Sum  Inputs=|++
  s_star : Outport
  wires:
  Sum1/1 -> Product1/2
  T/1 -> Product/1
  s_0/1 -> Sum/1
  Product1/1 -> Divide/1
  Product/1 -> Sum2/1
  Divide/1 -> Sum2/2
  x_dot_leader/1 -> Sum1/2
  Product2/1 -> Sqrt/1
  Sqrt/1 -> Gain/1
  Gain/1 -> Divide/2
  a/1 -> Product2/1
  b/1 -> Product2/2
  Constant/1 -> Max/2
  Sum2/1 -> Max/1
  Max/1 -> Sum/2
  Sum/1 -> s_star/1
  x_dot_follower/1 -> Product/2, Product1/1, Sum1/1

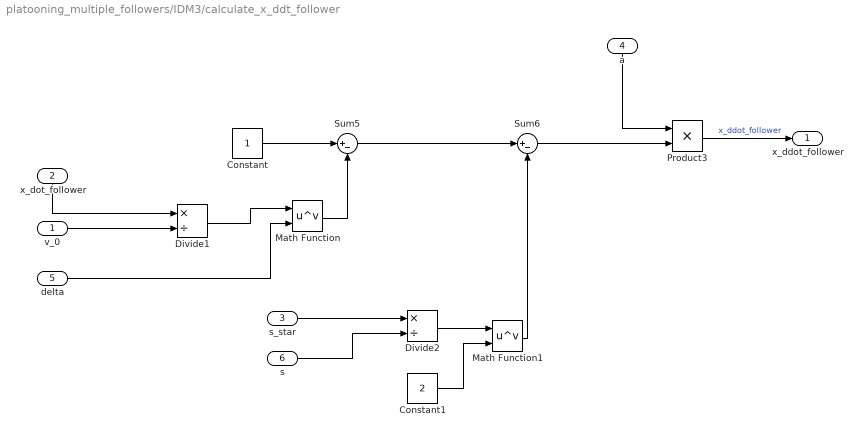
== system platooning_multiple_followers/IDM3/calculate_x_ddt_follower ==
  v_0 : Inport
  x_dot_follower : Inport  Port=2
  s_star : Inport  Port=3
  a : Inport  Port=4
  delta : Inport  Port=5
  s : Inport  Port=6
  Constant : Constant
  Constant1 : Constant  Value=2
  Divide1 : Product  Inputs=*/
  Divide2 : Product  Inputs=*/
  Math Function : Math  Operator=pow  SaturateOnIntegerOverflow=on
  Math Function1 : Math  Operator=pow  SaturateOnIntegerOverflow=on
  Product3 : Product
  Sum5 : Sum  Inputs=|+-
  Sum6 : Sum  Inputs=|+-
  x_ddot_follower : Outport
  wires:
  Product3/1 -> x_ddot_follower/1  "x_ddot_follower"
  v_0/1 -> Divide1/2
  Constant/1 -> Sum5/1
  Math Function/1 -> Sum5/2
  a/1 -> Product3/1
  x_dot_follower/1 -> Divide1/1
  s/1 -> Divide2/2
  s_star/1 -> Divide2/1
  Sum5/1 -> Sum6/1
  Constant1/1 -> Math Function1/2
  Divide1/1 -> Math Function/1
  Math Function1/1 -> Sum6/2
  delta/1 -> Math Function/2
  Divide2/1 -> Math Function1/1
  Sum6/1 -> Product3/2

== system platooning_multiple_followers/distance_check/If Action Subsystem2 ==
  time : Inport
  velocity : Inport  Port=2
  position : Inport  Port=3
  Action Port : ActionPort  ActionType=then
  CAN Pack : canmsglib/CAN Pack  MsgList=(none)  MsgName=CAN Msg  MsgIDType=Standard (11-bit identifier)  MsgIdentifier=1  MsgLength=8  SignalInfo=position$0$16$1$1$1$0$0.1$0$-Inf$Inf$#velocity$16$16$1$1$1$0$0.0025$0$-Inf$Inf$#timestamp$32$16$1$1$1$0$0.01$0$-Inf$Inf$#  NSignals=3  StartBits=str2num('[int32(0);int32(16);int32(32)]')  SignalSizes=str2num('[int32(16);int32(16);int32(16)]')  ByteOrders=str2num('[int32(1);int32(1);int32(1)]')  DataTypes=str2num('[int32(1);int32(1);int32(1)]')  MultiplexTypes=str2num('[int32(1);int32(1);int32(1)]')  MultiplexValues=str2num('[double(0);double(0);double(0)]')  Factors=str2num('[double(0.1);double(0.0025);double(0.01)]')  Offsets=str2num('[double(0);double(0);double(0)]')  Minimums=str2num('[double(-Inf);double(-Inf);double(-Inf)]')  Maximums=str2num('[double(Inf);double(Inf);double(Inf)]')  Remote=off  ApplyMinMax=off
      settings: SourceProductName=Simulink Real-Time  DataFormat=manually specified signals
  CAN Transmit1 : canlib/CAN Transmit  BlockHandle=569.0001  DeviceMenu=MathWorks Virtual 1 (Channel 1)  Device=MathWorks Virtual 1 (Channel 1)  ObjConstructor=canChannel('MathWorks','Virtual 1',1)  EnablePeriodicTransmit=off  MessagePeriod=1.000
      settings: SourceProductName=Vehicle Network Toolbox  SourceProductBaseCode=VN
  Data Store Write : DataStoreWrite  DataStoreName=t1
  Data Store Write1 : DataStoreWrite  DataStoreName=v1
  Data Store Write2 : DataStoreWrite  DataStoreName=x1
  wires:
  time/1 -> CAN Pack/3, Data Store Write/1
  velocity/1 -> CAN Pack/2, Data Store Write1/1
  CAN Pack/1 -> CAN Transmit1/1
  position/1 -> Data Store Write2/1, CAN Pack/1

== system platooning_multiple_followers/distance_check1/If Action Subsystem2 ==
  time : Inport
  velocity : Inport  Port=2
  position : Inport  Port=3
  Action Port : ActionPort  ActionType=then
  CAN Pack : canmsglib/CAN Pack  MsgList=(none)  MsgName=CAN Msg  MsgIDType=Standard (11-bit identifier)  MsgIdentifier=2  MsgLength=8  SignalInfo=position$0$16$1$1$1$0$0.1$0$-Inf$Inf$#velocity$16$16$1$1$1$0$0.0025$0$-Inf$Inf$#timestamp$32$16$1$1$1$0$0.01$0$-Inf$Inf$#  NSignals=3  StartBits=str2num('[int32(0);int32(16);int32(32)]')  SignalSizes=str2num('[int32(16);int32(16);int32(16)]')  ByteOrders=str2num('[int32(1);int32(1);int32(1)]')  DataTypes=str2num('[int32(1);int32(1);int32(1)]')  MultiplexTypes=str2num('[int32(1);int32(1);int32(1)]')  MultiplexValues=str2num('[double(0);double(0);double(0)]')  Factors=str2num('[double(0.1);double(0.0025);double(0.01)]')  Offsets=str2num('[double(0);double(0);double(0)]')  Minimums=str2num('[double(-Inf);double(-Inf);double(-Inf)]')  Maximums=str2num('[double(Inf);double(Inf);double(Inf)]')  Remote=off  ApplyMinMax=off
      settings: SourceProductName=Simulink Real-Time  DataFormat=manually specified signals
  CAN Transmit1 : canlib/CAN Transmit  BlockHandle=610.0001  DeviceMenu=MathWorks Virtual 1 (Channel 1)  Device=MathWorks Virtual 1 (Channel 1)  ObjConstructor=canChannel('MathWorks','Virtual 1',1)  EnablePeriodicTransmit=off  MessagePeriod=1.000
      settings: SourceProductName=Vehicle Network Toolbox  SourceProductBaseCode=VN
  Data Store Write : DataStoreWrite  DataStoreName=t2
  Data Store Write1 : DataStoreWrite  DataStoreName=v2
  Data Store Write2 : DataStoreWrite  DataStoreName=x2
  wires:
  time/1 -> CAN Pack/3, Data Store Write/1
  velocity/1 -> CAN Pack/2, Data Store Write1/1
  CAN Pack/1 -> CAN Transmit1/1
  position/1 -> Data Store Write2/1, CAN Pack/1

== system platooning_multiple_followers/distance_check2/If Action Subsystem2 ==
  time : Inport
  velocity : Inport  Port=2
  position : Inport  Port=3
  Action Port : ActionPort  ActionType=then
  CAN Pack : canmsglib/CAN Pack  MsgList=(none)  MsgName=CAN Msg  MsgIDType=Standard (11-bit identifier)  MsgIdentifier=3  MsgLength=8  SignalInfo=position$0$16$1$1$1$0$0.1$0$-Inf$Inf$#velocity$16$16$1$1$1$0$0.0025$0$-Inf$Inf$#timestamp$32$16$1$1$1$0$0.01$0$-Inf$Inf$#  NSignals=3  StartBits=str2num('[int32(0);int32(16);int32(32)]')  SignalSizes=str2num('[int32(16);int32(16);int32(16)]')  ByteOrders=str2num('[int32(1);int32(1);int32(1)]')  DataTypes=str2num('[int32(1);int32(1);int32(1)]')  MultiplexTypes=str2num('[int32(1);int32(1);int32(1)]')  MultiplexValues=str2num('[double(0);double(0);double(0)]')  Factors=str2num('[double(0.1);double(0.0025);double(0.01)]')  Offsets=str2num('[double(0);double(0);double(0)]')  Minimums=str2num('[double(-Inf);double(-Inf);double(-Inf)]')  Maximums=str2num('[double(Inf);double(Inf);double(Inf)]')  Remote=off  ApplyMinMax=off
      settings: SourceProductName=Simulink Real-Time  DataFormat=manually specified signals
  CAN Transmit1 : canlib/CAN Transmit  BlockHandle=651.0001  DeviceMenu=MathWorks Virtual 1 (Channel 1)  Device=MathWorks Virtual 1 (Channel 1)  ObjConstructor=canChannel('MathWorks','Virtual 1',1)  EnablePeriodicTransmit=off  MessagePeriod=1.000
      settings: SourceProductName=Vehicle Network Toolbox  SourceProductBaseCode=VN
  Data Store Write : DataStoreWrite  DataStoreName=t3
  Data Store Write1 : DataStoreWrite  DataStoreName=v3
  Data Store Write2 : DataStoreWrite  DataStoreName=x3
  wires:
  time/1 -> CAN Pack/3, Data Store Write/1
  velocity/1 -> CAN Pack/2, Data Store Write1/1
  CAN Pack/1 -> CAN Transmit1/1
  position/1 -> Data Store Write2/1, CAN Pack/1

== system platooning_multiple_followers/distance_check3/If Action Subsystem2 ==
  time : Inport
  velocity : Inport  Port=2
  position : Inport  Port=3
  Action Port : ActionPort  ActionType=then
  CAN Pack : canmsglib/CAN Pack  MsgList=(none)  MsgName=CAN Msg  MsgIDType=Standard (11-bit identifier)  MsgIdentifier=4  MsgLength=8  SignalInfo=position$0$16$1$1$1$0$0.1$0$-Inf$Inf$#velocity$16$16$1$1$1$0$0.0025$0$-Inf$Inf$#timestamp$32$16$1$1$1$0$0.01$0$-Inf$Inf$#  NSignals=3  StartBits=str2num('[int32(0);int32(16);int32(32)]')  SignalSizes=str2num('[int32(16);int32(16);int32(16)]')  ByteOrders=str2num('[int32(1);int32(1);int32(1)]')  DataTypes=str2num('[int32(1);int32(1);int32(1)]')  MultiplexTypes=str2num('[int32(1);int32(1);int32(1)]')  MultiplexValues=str2num('[double(0);double(0);double(0)]')  Factors=str2num('[double(0.1);double(0.0025);double(0.01)]')  Offsets=str2num('[double(0);double(0);double(0)]')  Minimums=str2num('[double(-Inf);double(-Inf);double(-Inf)]')  Maximums=str2num('[double(Inf);double(Inf);double(Inf)]')  Remote=off  ApplyMinMax=off
      settings: SourceProductName=Simulink Real-Time  DataFormat=manually specified signals
  CAN Transmit1 : canlib/CAN Transmit  BlockHandle=692.0001  DeviceMenu=MathWorks Virtual 1 (Channel 1)  Device=MathWorks Virtual 1 (Channel 1)  ObjConstructor=canChannel('MathWorks','Virtual 1',1)  EnablePeriodicTransmit=off  MessagePeriod=1.000
      settings: SourceProductName=Vehicle Network Toolbox  SourceProductBaseCode=VN
  Data Store Write : DataStoreWrite  DataStoreName=t4
  Data Store Write1 : DataStoreWrite  DataStoreName=v4
  Data Store Write2 : DataStoreWrite  DataStoreName=x4
  wires:
  time/1 -> CAN Pack/3, Data Store Write/1
  velocity/1 -> CAN Pack/2, Data Store Write1/1
  CAN Pack/1 -> CAN Transmit1/1
  position/1 -> Data Store Write2/1, CAN Pack/1
